simulink model "parteA"  (R2022b)
settings: Solver=VariableStepAuto  StartTime=0.0  StopTime=300  RelTol=1e-3
libraries: fuzblock x1, simulink x1
settings Model: Creator=andre  LastModifiedBy=maria
settings SolverCC: AlgebraicLoopSolver=TrustRegion
settings DebuggingCC: UnconnectedInputMsg=warning  UnconnectedOutputMsg=warning  UnconnectedLineMsg=warning  SFMachineParentedDataDiag=warning
settings ModelReferenceCC: EnableRefExpFcnMdlSchedulingChecks=on
settings RTWCC: DLArmComputeVersion=19.05

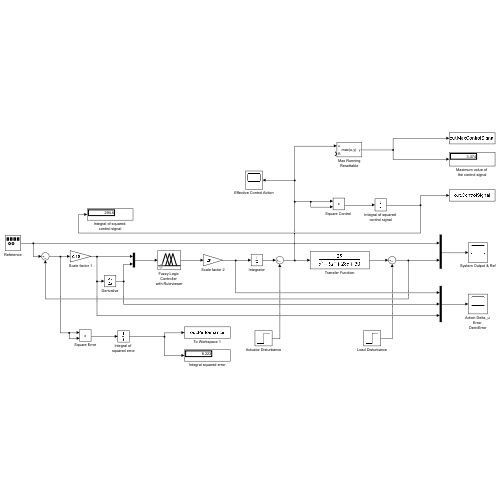
[thumbnail: Simulink's stored preview of the top-level diagram]
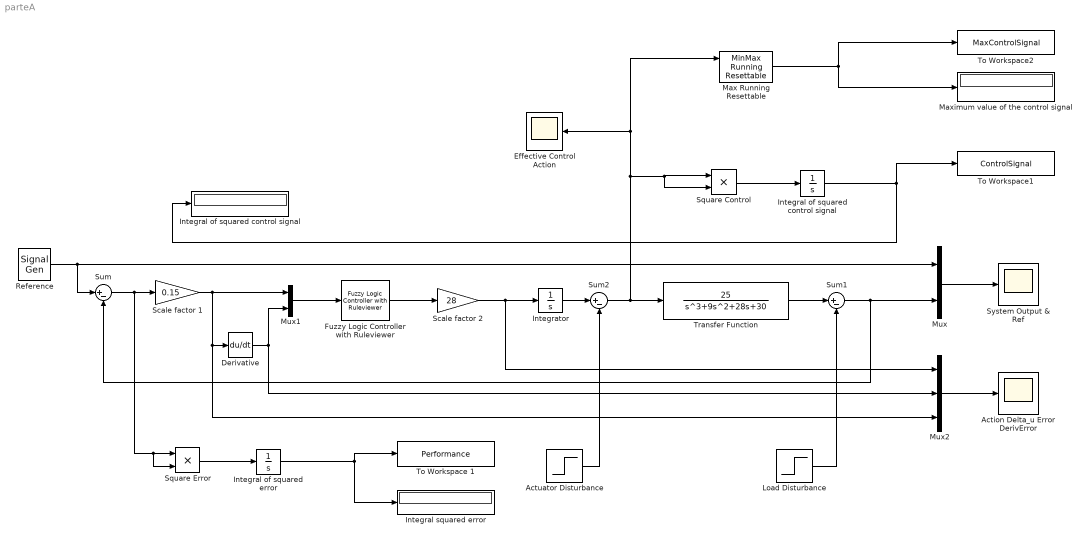
== system parteA ==
  Action Delta_u Error DerivError : Scope
  Actuator Disturbance : Step  Time=100  SampleTime=0
  Derivative : Derivative
  Effective Control Action : Scope
  Fuzzy Logic Controller with Ruleviewer : fuzblock/Fuzzy Logic  Controller  with Ruleviewer  fismatrix=sugeno_25_gauss  Ts=1
  Integral of squared error : Integrator
  Integral of squared control signal : Display
  "Integral of squared control signal " : Integrator
  Integral squared error : Display
  Integrator : Integrator
  Load Disturbance : Step  Time=200  SampleTime=0
  Max Running Resettable : simulink/Math Operations/MinMax Running Resettable  Function=max  vinit=0.0
  Maximum value of the control signal : Display
  Mux : Mux  Inputs=2
  Mux1 : Mux  Inputs=2
  Mux2 : Mux  Inputs=3
  Reference : SignalGenerator  WaveForm=sawtooth  Frequency=0.05  Units=rad/sec
  Scale factor 1 : Gain  Gain=0.15
  Scale factor 2 : Gain  Gain=28
  "Square Control " : Product
  Square Error : Product
  Sum : Sum  Inputs=|+-
  Sum1 : Sum  Inputs=|+-
  Sum2 : Sum  Inputs=|+-
  System Output & Ref : Scope
  To Workspace 1 : ToWorkspace  VariableName=Performance  SaveFormat=Timeseries  SampleTime=-1
  To Workspace1 : ToWorkspace  VariableName=ControlSignal  SaveFormat=Timeseries  SampleTime=-1
  To Workspace2 : ToWorkspace  VariableName=MaxControlSignal  SaveFormat=Timeseries  SampleTime=-1
  Transfer Function : TransferFcn  Numerator=[25]  Denominator=[1 9 28 30]
  wires:
  Reference/1 -> Sum/1, Mux/1
  Sum/1 -> Scale factor 1/1, Square Error/2, Square Error/1
  Mux1/1 -> Fuzzy Logic Controller with Ruleviewer/1
  Fuzzy Logic Controller with Ruleviewer/1 -> Scale factor 2/1
  Scale factor 1/1 -> Mux2/3, Derivative/1, Mux1/1
  Square Error/1 -> Integral of squared error/1
  Integral of squared error/1 -> Integral squared error/1, To Workspace 1/1
  Scale factor 2/1 -> Integrator/1, Mux2/1
  Integrator/1 -> Sum2/1
  Sum2/1 -> Transfer Function/1, Max Running Resettable/1, Effective Control Action/1, "Square Control "/2, "Square Control "/1
  Transfer Function/1 -> Sum1/1
  Mux/1 -> System Output & Ref/1
  Mux2/1 -> Action Delta_u Error DerivError/1
  Derivative/1 -> Mux2/2, Mux1/2
  Sum1/1 -> Mux/2, Sum/2
  "Square Control "/1 -> "Integral of squared control signal "/1
  "Integral of squared control signal "/1 -> Integral of squared control signal/1, To Workspace1/1
  Max Running Resettable/1 -> Maximum value of the control signal/1, To Workspace2/1
  Actuator Disturbance/1 -> Sum2/2
  Load Disturbance/1 -> Sum1/2
